simulink model "lab4_0"  (R2020b)
settings: Solver=VariableStepAuto  StartTime=0.0  StopTime=10  RelTol=1e-3
model workspace (MAT data in the model file):
  A = 0.5
  kd = 60
  ki = 60
  kp = 60
settings Model: Creator=Dexp  LastModifiedBy=takem

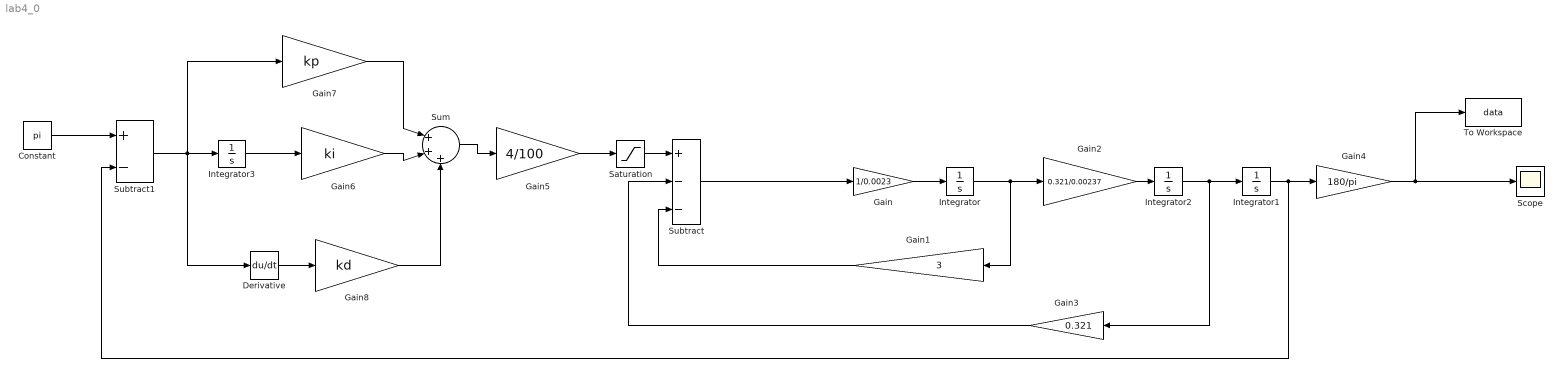
== system lab4_0 ==
  Constant : Constant  Value=pi
  Derivative : Derivative
  Gain : Gain  Gain=1/0.0023
  Gain1 : Gain  Gain=3
  Gain2 : Gain  Gain=0.321/0.00237
  Gain3 : Gain  Gain=0.321
  Gain4 : Gain  Gain=180/pi
  Gain5 : Gain  Gain=4/100
  Gain6 : Gain  Gain=ki
  Gain7 : Gain  Gain=kp
  Gain8 : Gain  Gain=kd
  Integrator : Integrator
  Integrator1 : Integrator
  Integrator2 : Integrator
  Integrator3 : Integrator  LimitOutput=on  UpperSaturationLimit=A  LowerSaturationLimit=-A
  Saturation : Saturate  UpperLimit=4  LowerLimit=-4
  Scope : Scope
  Subtract : Sum  Inputs=+--
  Subtract1 : Sum  Inputs=+-
  Sum : Sum  Inputs=|+++
  To Workspace : ToWorkspace  VariableName=data  SampleTime=-1
      settings: Save2DSignal=2-D array (concatenate along first dimension)
  wires:
  Constant/1 -> Subtract1/1
  Gain2/1 -> Integrator2/1
  Gain/1 -> Integrator/1
  Gain1/1 -> Subtract/3
  Gain3/1 -> Subtract/2
  Integrator2/1 -> Gain3/1, Integrator1/1
  Subtract/1 -> Gain/1
  Saturation/1 -> Subtract/1
  Integrator1/1 -> Subtract1/2, Gain4/1
  Integrator/1 -> Gain2/1, Gain1/1
  Gain4/1 -> To Workspace/1, Scope/1
  Gain5/1 -> Saturation/1
  Sum/1 -> Gain5/1
  Subtract1/1 -> Gain7/1, Derivative/1, Integrator3/1
  Integrator3/1 -> Gain6/1
  Gain6/1 -> Sum/2
  Derivative/1 -> Gain8/1
  Gain8/1 -> Sum/3
  Gain7/1 -> Sum/1
